simulink model "CM455A_Tauj0CfgAndUse"  (R2013b)
settings: Solver=FixedStepDiscrete  SolverMode=SingleTasking  StartTime=0.0  StopTime=1  FixedStep=0.0005  RelTol=1e-3
values from neighbouring files (symbols this model uses):
  PHAONTIMEASDMAX_NANOSEC_U32 = DataDict.Constant    [CM455A_Tauj0CfgAndUse_DataDict.m]
  TAUJ0TIPERCNT_NANOSECPERCNT_U15P1 = DataDict.Constant    [CM455A_Tauj0CfgAndUse_DataDict.m]
undefined symbols (not defined in the file or in its folder): sigbuilder_block
libraries: simulink x3, NxtrLim x3
settings Model: ModifiedHistory=Rev 008: Updated model to Matlab 2013B, added comments to show requirement linkage  Creator=nz3zln  LastModifiedBy=FZG88Y
settings SolverCC: AutoInsertRateTranBlk=on  InsertRTBMode=Always
settings DataIOCC: LimitDataPoints=off  SaveFormat=Structure  ReturnWorkspaceOutputs=on
settings OptimizationCC: BlockReduction=off  InlineParams=on  ZeroExternalMemoryAtStartup=off  ZeroInternalMemoryAtStartup=off  OptimizeModelRefInitCode=on  LifeSpan=1
settings DebuggingCC: SignalInfNanChecking=error  SignalRangeChecking=warning  UnderspecifiedInitializationDetection=Simplified  SolverPrmCheckMsg=error  InheritedTsInSrcMsg=error  DiscreteInheritContinuousMsg=error  SingleTaskRateTransMsg=error  TasksWithSamePriorityMsg=error  SigSpecEnsureSampleTimeMsg=error  CheckMatrixSingularityMsg=error  ParameterUnderflowMsg=error  ParameterPrecisionLossMsg=error  ParameterTunabilityLossMsg=error  FixptConstUnderflowMsg=warning  FixptConstOverflowMsg=warning  VectorMatrixConversionMsg=error  SignalLabelMismatchMsg=error  UnconnectedInputMsg=error  UnconnectedOutputMsg=error  UnconnectedLineMsg=error  SFcnCompatibilityMsg=error  UniqueDataStoreMsg=warning  BusObjectLabelMismatch=error  RootOutportRequireBusObject=error  AssertControl=DisableAll  ModelReferenceIOMsg=error  ModelReferenceVersionMismatchMessage=warning  ModelReferenceIOMismatchMessage=error  ModelReferenceCSMismatchMessage=warning  ModelReferenceDataLoggingMessage=error  StateNameClashWarn=warning  StrictBusMsg=ErrorOnBusTreatedAsVector  NonBusSignalsTreatedAsBus=error  SFUnexpectedBacktrackingDiag=error  SFInvalidInputDataAccessInChartInitDiag=error  SFNoUnconditionalDefaultTransitionDiag=error  SFTransitionOutsideNaturalParentDiag=error  SFUnconditionalTransitionShadowingDiag=error  SFUndirectedBroadcastEventsDiag=error
settings ModelReferenceCC: ModelReferenceNumInstancesAllowed=Single
settings RTWCC: SystemTargetFile=autosar.tlc  GenCodeOnly=on  TemplateMakefile=ert_default_tmf  Description=AUTOSAR  GenerateReport=on  ProcessScript=autosar_make_rtw_hook  LaunchReport=on
settings CodeAppCC: GenerateComments=off  IgnoreCustomStorageClasses=off  CustomSymbolStrType=$N$R$M  CustomSymbolStrBlkIO=$N$M  SimulinkBlockComments=off
settings STFCustomTargetCC: ParMdlRefBuildCompliant=on  CompOptLevelCompliant=on  IncludeMdlTerminateFcn=off  CombineOutputUpdateFcns=on  SuppressErrorStatus=on  ERTFirstTimeCompliant=on  ERTCustomFileBanners=on  SupportNonFinite=off  SupportComplex=off  SupportContinuousTime=off  SupportNonInlinedSFcns=off  MATLABClassNameForMDSCustomization=Simulink.SoftwareTarget.ERTCustomization  AutosarCompliant=on  GRTInterface=off  SystemTargetFile=autosar.tlc
settings ERTTargetCC: CodeReplacementLibrary=ANSI_C  ConcurrentExecutionCompliant=off  IncludeMdlTerminateFcn=off  SuppressErrorStatus=on  SupportNonFinite=off  SupportComplex=off  ModelStepFunctionPrototypeControlCompliant=off  CPPClassGenCompliant=off  AutosarCompliant=on  InlinedParameterPlacement=NonHierarchical  ERTCustomFileTemplate=example_file_process.tlc  EnableUserReplacementTypes=on

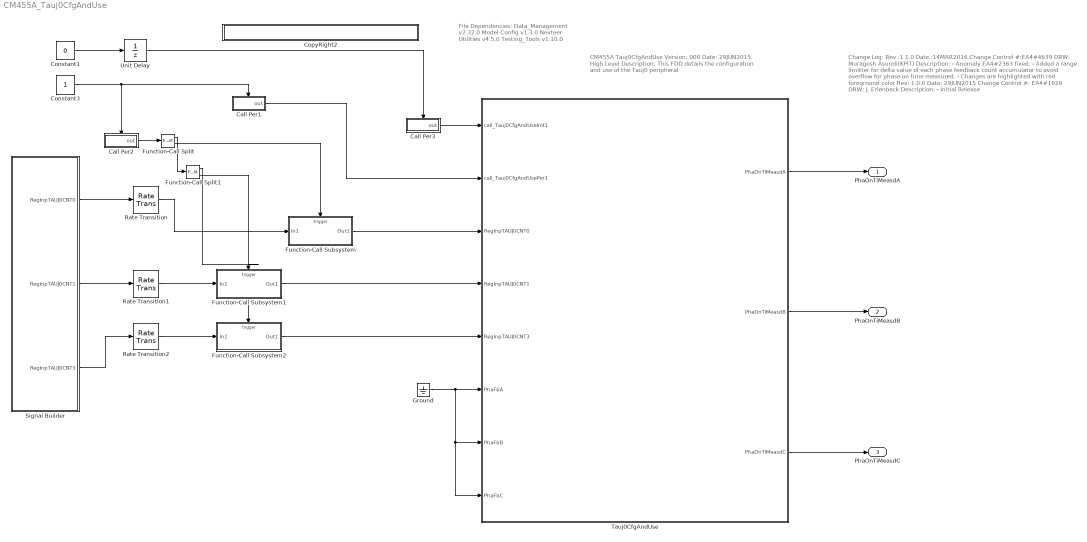
== system CM455A_Tauj0CfgAndUse ==
  note: CM455A Tauj0CfgAndUse
      |
      | Version: 000
      | Date: 29JUN2015
      |
      | High Level Description:
      | This FDD details the configuration and use of the Tauj0
      | peripheral
  note: Change Log:
      | Rev :1.1.0
      | Date :14MAR2016
      | Change Control #:EA4#4639
      | DRW: Muragesh Asundi(KPIT)
      | Description:
      | - Anomaly EA4#2363 fixed.
      | - Added a range limitter for delta value of each phase
      |  feedback count accumulator to avoid overflow for phase on time measured.
      | - Changes are highlighted with red foreground color
      |
      | Rev: 1.0.0
      | Date: 29JUN2015
      | Change Control #: EA4#1928
      | DRW: J. Erlenbeck
      | Description:
      | - Initial Release
  note: File Dependencies:
      | Data_Management v2.32.0
      | Model Config v1.3.0
      | Nexteer Utilities v4.5.0
      | Testing_Tools v1.10.0
  Call Per1 : Subsystem  TreatAsAtomicUnit=on
  Call Per2 : Subsystem  TreatAsAtomicUnit=on
  Call Per3 : Subsystem  TreatAsAtomicUnit=on
  Constant1 : Constant  Value=0  OutDataTypeStr=int8
  Constant3 : Constant  OutDataTypeStr=int8
  CopyRight2 : Subsystem  Description=|  mask(Copyright Information){none=on}
      | Copyright info block.                                               
      |                                                                     
      | Place copyright information at the top of every subsystem in design.
      mask prompts: none "No parameters"
      mask help: Place copyright information at the top of every subsystem in design.
      mask Display:
      | NxtrConf = 'Nexteer Confidential';
      | 
      | sys = bdroot; %handle for the current model ("system")
      | first = get_param(sys,'Created');
      | first = first(end-3:end);  %year is last four digits
      | 
      | last = get_param(sys,'LastModifiedDate');
      | if isempty(last)
      |     last = datestr(now,'yyyy');
      | else
      |     last = last(end-3:end);
      | end
      | 
      | if strcmp(first,last)
      |     fprintf('%s -- Copyright %s Nexteer',NxtrConf,first)
      | else
      |     fprintf('%s -- %s%s- %s Nexteer',NxtrConf,char(169),first,last)
      | end
  Function-Call Split : FunctionCallSplit
  Function-Call Split1 : FunctionCallSplit
  Function-Call Subsystem : Subsystem  TreatAsAtomicUnit=on
  Function-Call Subsystem1 : Subsystem  TreatAsAtomicUnit=on
  Function-Call Subsystem2 : Subsystem  TreatAsAtomicUnit=on
  Ground : Ground
  Rate Transition : RateTransition
  Rate Transition1 : RateTransition
  Rate Transition2 : RateTransition
  Signal Builder : Subsystem  Tag=STV Subsys  LoadFcn=sigbuilder_block('load');  StartFcn=sigbuilder_block('start');  StopFcn=sigbuilder_block('stop');  ClipboardFcn=sigbuilder_block('clipboard');  mask(Sigbuilder block){}
      mask help: Simulink:masks:SigbuilderBlock_MD
      mask init:
      | if ~strcmp(get_param(bdroot(gcbh),'SimulationStatus'),'stopped') tuvar = sigbuilder_block('maskInit'); end
      settings: CopyFcn=sigbuilder_block('copy');  DeleteFcn=sigbuilder_block('delete');  ModelCloseFcn=sigbuilder_block('modelClose');  PreSaveFcn=sigbuilder_block('preSave');  PauseFcn=sigbuilder_block('pause');  ContinueFcn=sigbuilder_block('continue');  NameChangeFcn=sigbuilder_block('namechange');  OpenFcn=sigbuilder_block('open',[0 124.5 635.25 388.5 ]);  CloseFcn=sigbuilder_block('close');
      mask Display: plot(0, 0, 100, 100,[2, 2, 32, 32, 2], [68, 8, 8, 68, 68],[32, 2], [38, 38], [32, 19, 2],[53, 60, 44], [32, 17, 17, 2],[16, 16, 31, 31]);txt = getActiveGroup(gcbh);text(2, 100, txt,'verticalAlignment', 'top');
  Tauj0CfgAndUse : Subsystem
  Unit Delay : UnitDelay  InitialCondition=1  SampleTime=-1
  PhaOnTiMeasdA : Outport
  PhaOnTiMeasdB : Outport  Port=2
  PhaOnTiMeasdC : Outport  Port=3
  wires:
  Constant3/1 -> Call Per2/Enable, Call Per1/Enable
  Signal Builder/1(RegInpTAUJ0CNT0) -> Rate Transition/1
  Call Per1/1(out) -> Tauj0CfgAndUse/2(call_Tauj0CfgAndUsePer1)
  Function-Call Subsystem/1(Out1) -> Tauj0CfgAndUse/3(RegInpTAUJ0CNT0)
  Rate Transition/1 -> Function-Call Subsystem/1(In1)
  Signal Builder/2(RegInpTAUJ0CNT1) -> Rate Transition1/1
  Signal Builder/3(RegInpTAUJ0CNT3) -> Rate Transition2/1
  Rate Transition1/1 -> Function-Call Subsystem1/1(In1)
  Rate Transition2/1 -> Function-Call Subsystem2/1(In1)
  Call Per2/1(out) -> Function-Call Split/1
  Function-Call Split/2 -> Function-Call Subsystem/Trigger
  Function-Call Split/1 -> Function-Call Split1/1
  Function-Call Split1/2 -> Function-Call Subsystem1/Trigger
  Function-Call Split1/1 -> Function-Call Subsystem2/Trigger
  Function-Call Subsystem1/1(Out1) -> Tauj0CfgAndUse/4(RegInpTAUJ0CNT1)
  Function-Call Subsystem2/1(Out1) -> Tauj0CfgAndUse/5(RegInpTAUJ0CNT3)
  Constant1/1 -> Unit Delay/1
  Unit Delay/1 -> Call Per3/Enable
  Call Per3/1(out) -> Tauj0CfgAndUse/1(call_Tauj0CfgAndUseInit1)
  Ground/1 -> Tauj0CfgAndUse/8(PhaFbC), Tauj0CfgAndUse/7(PhaFbB), Tauj0CfgAndUse/6(PhaFbA)
  Tauj0CfgAndUse/1(PhaOnTiMeasdA) -> PhaOnTiMeasdA/1
  Tauj0CfgAndUse/2(PhaOnTiMeasdB) -> PhaOnTiMeasdB/1
  Tauj0CfgAndUse/3(PhaOnTiMeasdC) -> PhaOnTiMeasdC/1

== system CM455A_Tauj0CfgAndUse/Call Per1 ==
  Enable : EnablePort
  Function Call Trigger : simulink/Ports & Subsystems/Function-Call Generator  RequirementInfo={} %GIDa_6dd05ab1_f91b_4d7a_a0ec_1170d213fa7b  sample_time=0.002  numberOfIterations=1
  out : Outport
  wires:
  Function Call Trigger/1 -> out/1

== system CM455A_Tauj0CfgAndUse/Call Per2 ==
  Enable : EnablePort
  Function Call Trigger : simulink/Ports & Subsystems/Function-Call Generator  RequirementInfo={} %GIDa_ae766dae_e1c3_424a_a7dd_99da62b4e21f  sample_time=0.0005  numberOfIterations=1
  out : Outport
  wires:
  Function Call Trigger/1 -> out/1

== system CM455A_Tauj0CfgAndUse/Call Per3 ==
  Enable : EnablePort
  Function Call Trigger : simulink/Ports & Subsystems/Function-Call Generator  RequirementInfo={} %GIDa_4dbf052b_4973_407d_b675_b3a9817a3516  sample_time=0.002  numberOfIterations=1
  out : Outport
  wires:
  Function Call Trigger/1 -> out/1

== system CM455A_Tauj0CfgAndUse/CopyRight2 ==

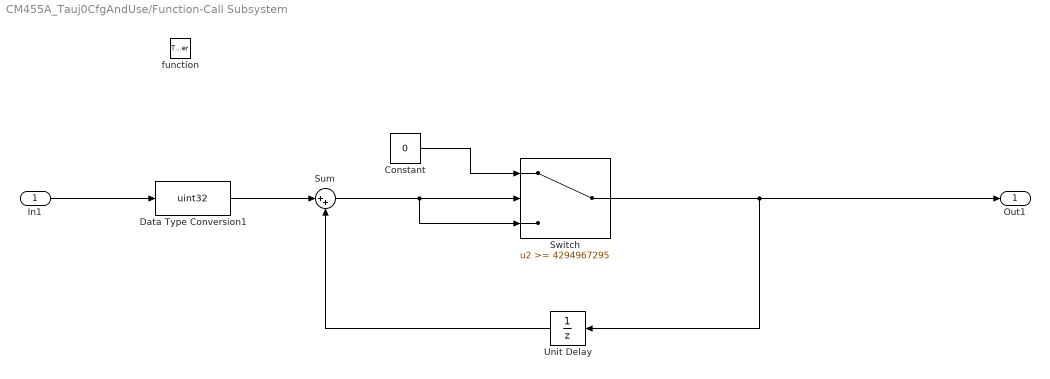
== system CM455A_Tauj0CfgAndUse/Function-Call Subsystem ==
  In1 : Inport
  function : TriggerPort  TriggerType=function-call
  Constant : Constant  Value=0  OutDataTypeStr=uint16
  Data Type Conversion1 : DataTypeConversion  OutDataTypeStr=uint32  RndMeth=Nearest
  Sum : Sum  Inputs=|++
  Switch : Switch  Threshold=4294967295
  Unit Delay : UnitDelay  SampleTime=-1
  Out1 : Outport
  wires:
  Constant/1 -> Switch/1
  Sum/1 -> Switch/3, Switch/2
  Data Type Conversion1/1 -> Sum/1
  Switch/1 -> Out1/1, Unit Delay/1
  Unit Delay/1 -> Sum/2
  In1/1 -> Data Type Conversion1/1

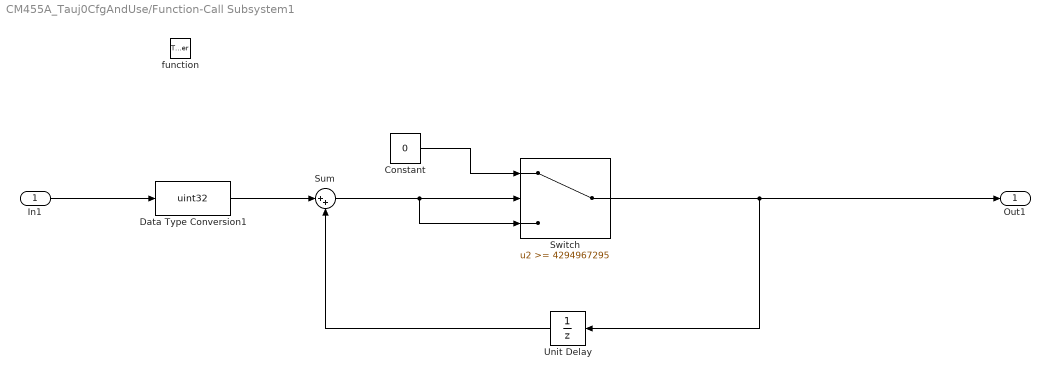
== system CM455A_Tauj0CfgAndUse/Function-Call Subsystem1 ==
  In1 : Inport
  function : TriggerPort  TriggerType=function-call
  Constant : Constant  Value=0  OutDataTypeStr=uint16
  Data Type Conversion1 : DataTypeConversion  OutDataTypeStr=uint32  RndMeth=Nearest
  Sum : Sum  Inputs=|++
  Switch : Switch  Threshold=4294967295
  Unit Delay : UnitDelay  SampleTime=-1
  Out1 : Outport
  wires:
  In1/1 -> Data Type Conversion1/1
  Unit Delay/1 -> Sum/2
  Switch/1 -> Unit Delay/1, Out1/1
  Data Type Conversion1/1 -> Sum/1
  Sum/1 -> Switch/2, Switch/3
  Constant/1 -> Switch/1

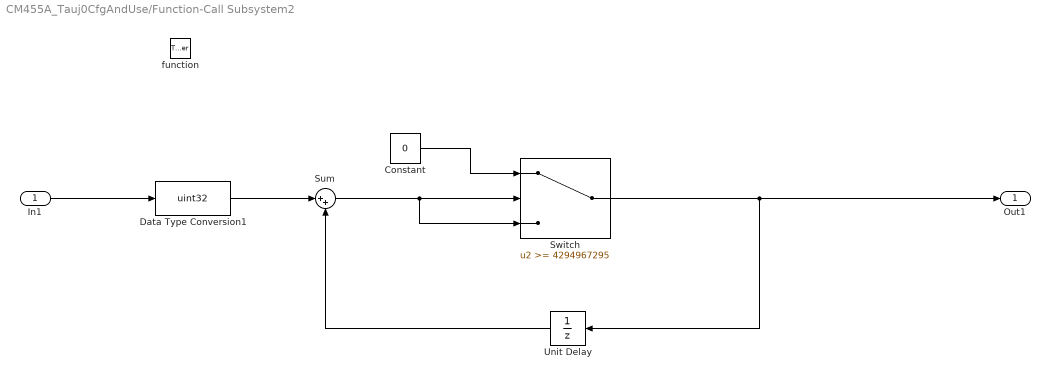
== system CM455A_Tauj0CfgAndUse/Function-Call Subsystem2 ==
  In1 : Inport
  function : TriggerPort  TriggerType=function-call
  Constant : Constant  Value=0  OutDataTypeStr=uint16
  Data Type Conversion1 : DataTypeConversion  OutDataTypeStr=uint32  RndMeth=Nearest
  Sum : Sum  Inputs=|++
  Switch : Switch  Threshold=4294967295
  Unit Delay : UnitDelay  SampleTime=-1
  Out1 : Outport
  wires:
  Constant/1 -> Switch/1
  Sum/1 -> Switch/3, Switch/2
  Data Type Conversion1/1 -> Sum/1
  Switch/1 -> Out1/1, Unit Delay/1
  Unit Delay/1 -> Sum/2
  In1/1 -> Data Type Conversion1/1

== system CM455A_Tauj0CfgAndUse/Signal Builder ==
  Demux : Demux  Tag=STV Demux  Outputs=3
  FromWs : FromWorkspace  Tag=STV FromWs  VariableName=tuvar  SampleTime=0
      SigBuilderData=|
      | common.afterFinalStr = 'Extrapolate'
      | common.sampleTime = 0
      | dataSet.timeRange = [0 2]
      | dataSet.name = 'Group 1'
      | sbobj.Groups.Name = 'Group 1'
      | sbobj.Groups.Signals(1).Name = 'RegInpTAUJ0CNT0'
      | sbobj.Groups.Signals(1).XData = [0 0.00125628140704 0.00251256281407 0.00376884422111 0.00502512562814 0.00628140703518 0.00753768844221 0.00879396984925 0.0100502512563 0.0113065326633 0.0125628140704 0.0138190954774 ... (1593 elements, 1x1593)]
      | sbobj.Groups.Signals(1).YData = [5000000 5157842.74882 5315528.15656 5472899.03897 5629798.52534 5786070.21484 5941558.33245 6096107.88424 6249564.81185 6401776.14609 6552590.15937 6701856.51702 ... (1593 elements, 1x1593)]
      | sbobj.Groups.Signals(2).Name = 'RegInpTAUJ0CNT1'
      | sbobj.Groups.Signals(2).XData = [0 0.5 0.5 1 1 1.5 1.5 2]
      | sbobj.Groups.Signals(2).YData = [0 4000000 0 4000000 0 4000000 0 4000000]
      | sbobj.Groups.Signals(3).Name = 'RegInpTAUJ0CNT3'
      | sbobj.Groups.Signals(3).XData = [0 0.0833333333333 0.0833333333333 0.2 0.2 0.416666666667 0.416666666667 0.514 0.514 0.966 0.966 1 1 1.298 1.298 1.33333333333 1.33333333333 1.598 1.598 1.66666666667 1.66666666667 1.946 1.946 2]
      | sbobj.Groups.Signals(3).YData = [10000000 10000000 0 0 10000000 10000000 0 0 10000000 10000000 0 0 10000000 10000000 0 0 10000000 10000000 0 0 10000000 10000000 0 0]
      | sbobj.Groups.TimeRange = [0 2]
  RegInpTAUJ0CNT0 : Outport  Tag=STV Outport
  RegInpTAUJ0CNT1 : Outport  Tag=STV Outport  Port=2
  RegInpTAUJ0CNT3 : Outport  Tag=STV Outport  Port=3
  wires:
  FromWs/1 -> Demux/1
  Demux/1 -> RegInpTAUJ0CNT0/1
  Demux/2 -> RegInpTAUJ0CNT1/1
  Demux/3 -> RegInpTAUJ0CNT3/1

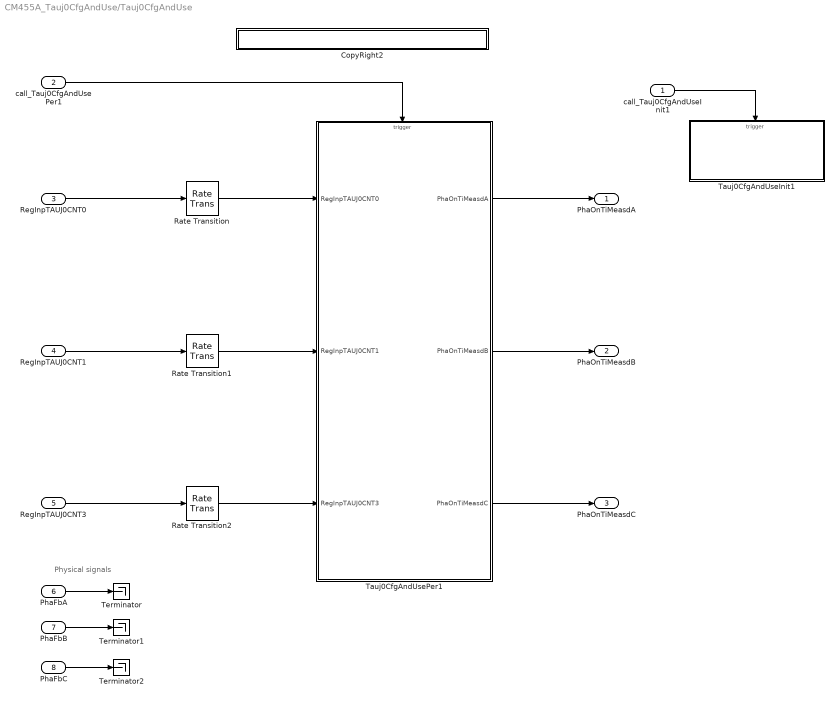
== system CM455A_Tauj0CfgAndUse/Tauj0CfgAndUse ==
  note: Physical signals
  call_Tauj0CfgAndUseInit1 : Inport  RequirementInfo={} %GIDa_c75e8815_b602_4250_97f2_eeb5dd1c39d1
  call_Tauj0CfgAndUsePer1 : Inport  RequirementInfo={} %GIDa_468d2479_6710_42ce_bd19_b69834ab6306  Port=2
  RegInpTAUJ0CNT0 : Inport  Port=3
  RegInpTAUJ0CNT1 : Inport  Port=4
  RegInpTAUJ0CNT3 : Inport  RequirementInfo={} %GIDa_84fb02b3_72b4_4e28_a17f_e99f7297de00  Port=5
  PhaFbA : Inport  Port=6
  PhaFbB : Inport  Port=7
  PhaFbC : Inport  Port=8
  CopyRight2 : Subsystem  Description=|  mask(Copyright Information){none=on}
      | Copyright info block.                                               
      |                                                                     
      | Place copyright information at the top of every subsystem in design.
      mask prompts: none "No parameters"
      mask help: Place copyright information at the top of every subsystem in design.
      mask Display:
      | NxtrConf = 'Nexteer Confidential';
      | 
      | sys = bdroot; %handle for the current model ("system")
      | first = get_param(sys,'Created');
      | first = first(end-3:end);  %year is last four digits
      | 
      | last = get_param(sys,'LastModifiedDate');
      | if isempty(last)
      |     last = datestr(now,'yyyy');
      | else
      |     last = last(end-3:end);
      | end
      | 
      | if strcmp(first,last)
      |     fprintf('%s -- Copyright %s Nexteer',NxtrConf,first)
      | else
      |     fprintf('%s -- %s%s- %s Nexteer',NxtrConf,char(169),first,last)
      | end
  Rate Transition : RateTransition
  Rate Transition1 : RateTransition
  Rate Transition2 : RateTransition
  Tauj0CfgAndUseInit1 : Subsystem  TreatAsAtomicUnit=on
  Tauj0CfgAndUsePer1 : Subsystem  TreatAsAtomicUnit=on
  Terminator : Terminator
  Terminator1 : Terminator
  Terminator2 : Terminator
  PhaOnTiMeasdA : Outport
  PhaOnTiMeasdB : Outport  Port=2
  PhaOnTiMeasdC : Outport  Port=3
  wires:
  call_Tauj0CfgAndUsePer1/1 -> Tauj0CfgAndUsePer1/Trigger
  RegInpTAUJ0CNT0/1 -> Rate Transition/1
  RegInpTAUJ0CNT1/1 -> Rate Transition1/1
  RegInpTAUJ0CNT3/1 -> Rate Transition2/1
  Rate Transition/1 -> Tauj0CfgAndUsePer1/1(RegInpTAUJ0CNT0)
  Rate Transition1/1 -> Tauj0CfgAndUsePer1/2(RegInpTAUJ0CNT1)
  Rate Transition2/1 -> Tauj0CfgAndUsePer1/3(RegInpTAUJ0CNT3)
  Tauj0CfgAndUsePer1/1(PhaOnTiMeasdA) -> PhaOnTiMeasdA/1
  Tauj0CfgAndUsePer1/2(PhaOnTiMeasdB) -> PhaOnTiMeasdB/1
  Tauj0CfgAndUsePer1/3(PhaOnTiMeasdC) -> PhaOnTiMeasdC/1
  call_Tauj0CfgAndUseInit1/1 -> Tauj0CfgAndUseInit1/Trigger
  PhaFbA/1 -> Terminator/1
  PhaFbB/1 -> Terminator1/1
  PhaFbC/1 -> Terminator2/1

== system CM455A_Tauj0CfgAndUse/Tauj0CfgAndUse/CopyRight2 ==

== system CM455A_Tauj0CfgAndUse/Tauj0CfgAndUse/Tauj0CfgAndUseInit1 ==
  note: Initialize the Tauj0 registers per
      | CM455A_Tauj0CfgAndUse_RegisterConfiguration.xlsm.  Initialize in order by row, top to bottom.
  function : TriggerPort  TriggerType=function-call
  CopyRight2 : Subsystem  Description=|  mask(Copyright Information){none=on}
      | Copyright info block.                                               
      |                                                                     
      | Place copyright information at the top of every subsystem in design.
      mask prompts: none "No parameters"
      mask help: Place copyright information at the top of every subsystem in design.
      mask Display:
      | NxtrConf = 'Nexteer Confidential';
      | 
      | sys = bdroot; %handle for the current model ("system")
      | first = get_param(sys,'Created');
      | first = first(end-3:end);  %year is last four digits
      | 
      | last = get_param(sys,'LastModifiedDate');
      | if isempty(last)
      |     last = datestr(now,'yyyy');
      | else
      |     last = last(end-3:end);
      | end
      | 
      | if strcmp(first,last)
      |     fprintf('%s -- Copyright %s Nexteer',NxtrConf,first)
      | else
      |     fprintf('%s -- %s%s- %s Nexteer',NxtrConf,char(169),first,last)
      | end

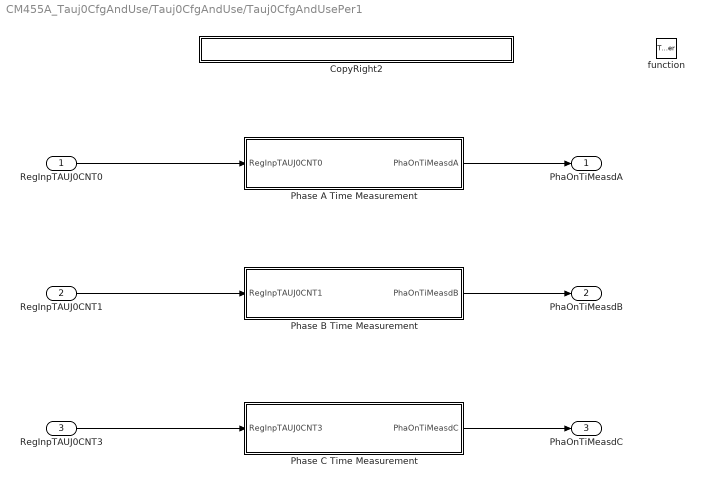
== system CM455A_Tauj0CfgAndUse/Tauj0CfgAndUse/Tauj0CfgAndUsePer1 ==
  RegInpTAUJ0CNT0 : Inport
  RegInpTAUJ0CNT1 : Inport  Port=2
  RegInpTAUJ0CNT3 : Inport  RequirementInfo={} %GIDa_d2e38bc4_d7b3_4726_bec9_8ac60b17d0ae  Port=3
  function : TriggerPort  TriggerType=function-call
  CopyRight2 : Subsystem  Description=|  mask(Copyright Information){none=on}
      | Copyright info block.                                               
      |                                                                     
      | Place copyright information at the top of every subsystem in design.
      mask prompts: none "No parameters"
      mask help: Place copyright information at the top of every subsystem in design.
      mask Display:
      | NxtrConf = 'Nexteer Confidential';
      | 
      | sys = bdroot; %handle for the current model ("system")
      | first = get_param(sys,'Created');
      | first = first(end-3:end);  %year is last four digits
      | 
      | last = get_param(sys,'LastModifiedDate');
      | if isempty(last)
      |     last = datestr(now,'yyyy');
      | else
      |     last = last(end-3:end);
      | end
      | 
      | if strcmp(first,last)
      |     fprintf('%s -- Copyright %s Nexteer',NxtrConf,first)
      | else
      |     fprintf('%s -- %s%s- %s Nexteer',NxtrConf,char(169),first,last)
      | end
  Phase A Time Measurement : Subsystem  RequirementInfo="{'linktype_rmi_doors' '0000cf4a (/ESG Group/FDD Module Requirements/EA4 Specific/CM455A_Tauj0CfgAndMeas)' '#CM455A_87' 'true' 'REQ:  CM455A_87' '' } %GIDa_7041a376_39d9_4031_9ce0_54f885feabcb"  TreatAsAtomicUnit=on
  Phase B Time Measurement : Subsystem  RequirementInfo="{'linktype_rmi_doors' '0000cf4a (/ESG Group/FDD Module Requirements/EA4 Specific/CM455A_Tauj0CfgAndMeas)' '#CM455A_95' 'true' 'REQ:  CM455A_95' '' } %GIDa_2958352a_abfa_49fb_ac22_38a600953ff5"  TreatAsAtomicUnit=on
  Phase C Time Measurement : Subsystem  RequirementInfo="{'linktype_rmi_doors' '0000cf4a (/ESG Group/FDD Module Requirements/EA4 Specific/CM455A_Tauj0CfgAndMeas)' '#CM455A_96' 'true' 'REQ:  CM455A_96' '' } %GIDa_b9e937c9_f0a4_435c_8980_887e05030cab"  TreatAsAtomicUnit=on
  PhaOnTiMeasdA : Outport
  PhaOnTiMeasdB : Outport  Port=2
  PhaOnTiMeasdC : Outport  Port=3
  wires:
  Phase A Time Measurement/1(PhaOnTiMeasdA) -> PhaOnTiMeasdA/1
  RegInpTAUJ0CNT0/1 -> Phase A Time Measurement/1(RegInpTAUJ0CNT0)
  Phase B Time Measurement/1(PhaOnTiMeasdB) -> PhaOnTiMeasdB/1
  RegInpTAUJ0CNT1/1 -> Phase B Time Measurement/1(RegInpTAUJ0CNT1)
  RegInpTAUJ0CNT3/1 -> Phase C Time Measurement/1(RegInpTAUJ0CNT3)
  Phase C Time Measurement/1(PhaOnTiMeasdC) -> PhaOnTiMeasdC/1

== system CM455A_Tauj0CfgAndUse/Tauj0CfgAndUse/Tauj0CfgAndUseInit1/CopyRight2 ==

== system CM455A_Tauj0CfgAndUse/Tauj0CfgAndUse/Tauj0CfgAndUsePer1/CopyRight2 ==

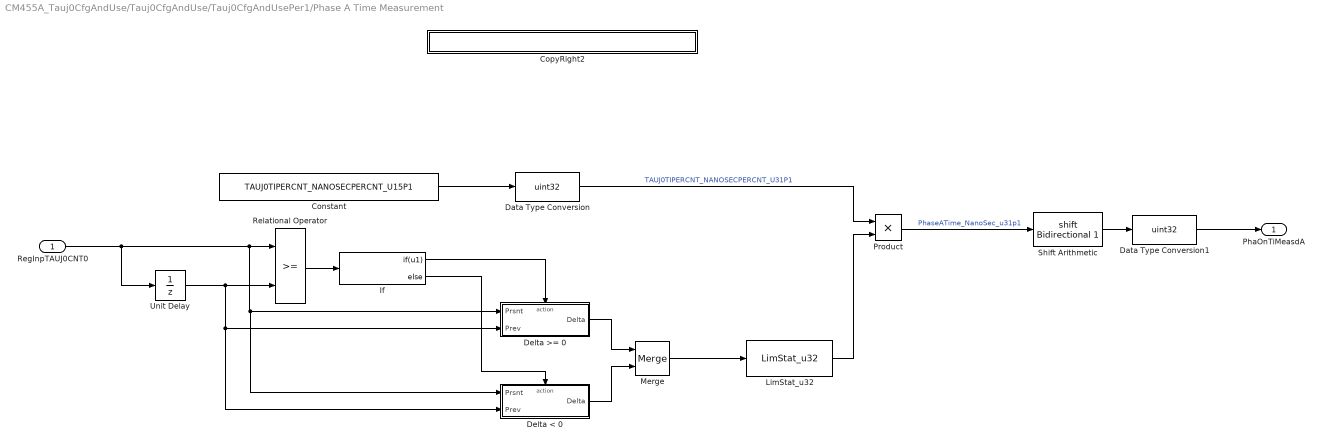
== system CM455A_Tauj0CfgAndUse/Tauj0CfgAndUse/Tauj0CfgAndUsePer1/Phase A Time Measurement ==
  RegInpTAUJ0CNT0 : Inport
  Constant : Constant  Value=TAUJ0TIPERCNT_NANOSECPERCNT_U15P1
  CopyRight2 : Subsystem  Description=|  mask(Copyright Information){none=on}
      | Copyright info block.                                               
      |                                                                     
      | Place copyright information at the top of every subsystem in design.
      mask prompts: none "No parameters"
      mask help: Place copyright information at the top of every subsystem in design.
      mask Display:
      | NxtrConf = 'Nexteer Confidential';
      | 
      | sys = bdroot; %handle for the current model ("system")
      | first = get_param(sys,'Created');
      | first = first(end-3:end);  %year is last four digits
      | 
      | last = get_param(sys,'LastModifiedDate');
      | if isempty(last)
      |     last = datestr(now,'yyyy');
      | else
      |     last = last(end-3:end);
      | end
      | 
      | if strcmp(first,last)
      |     fprintf('%s -- Copyright %s Nexteer',NxtrConf,first)
      | else
      |     fprintf('%s -- %s%s- %s Nexteer',NxtrConf,char(169),first,last)
      | end
  Data Type Conversion : DataTypeConversion  OutDataTypeStr=uint32
  Data Type Conversion1 : DataTypeConversion  OutDataTypeStr=uint32
  Delta < 0 : Subsystem  TreatAsAtomicUnit=on
  Delta >= 0 : Subsystem  TreatAsAtomicUnit=on
  If : If  IfExpression=u1
  LimStat_u32 : NxtrLim/LimStat_u32  LoLim=PHAFBDELTACNTMIN_CNT_U32  HiLim=PHAFBDELTACNTMAX_CNT_U32
      settings: AttributesFormatString=|
      | Low Limit: %<LoLim>
      | High Limit:%<HiLim>
  Merge : Merge
  Product : Product
  Relational Operator : RelationalOperator  OutDataTypeStr=boolean
  Shift Arithmetic : ArithShift  BitShiftNumber=1
  Unit Delay : UnitDelay  SampleTime=-1  StateName=PhaOnTiCntrAPrev  StateMustResolveToSignalObject=on
      settings: AttributesFormatString=|
      | State Variable:
      | %<StateName>
  PhaOnTiMeasdA : Outport
  wires:
  Unit Delay/1 -> Delta < 0/2(Prev), Delta >= 0/2(Prev), Relational Operator/2
  Constant/1 -> Data Type Conversion/1
  Data Type Conversion/1 -> Product/1  "TAUJ0TIPERCNT_NANOSECPERCNT_U31P1"
  Shift Arithmetic/1 -> Data Type Conversion1/1
  Data Type Conversion1/1 -> PhaOnTiMeasdA/1
  RegInpTAUJ0CNT0/1 -> Delta < 0/1(Prsnt), Delta >= 0/1(Prsnt), Relational Operator/1, Unit Delay/1
  Product/1 -> Shift Arithmetic/1  "PhaseATime_NanoSec_u31p1"
  Relational Operator/1 -> If/1
  If/1 -> Delta >= 0/Action
  If/2 -> Delta < 0/Action
  LimStat_u32/1 -> Product/2
  Delta >= 0/1(Delta) -> Merge/1
  Delta < 0/1(Delta) -> Merge/2
  Merge/1 -> LimStat_u32/1

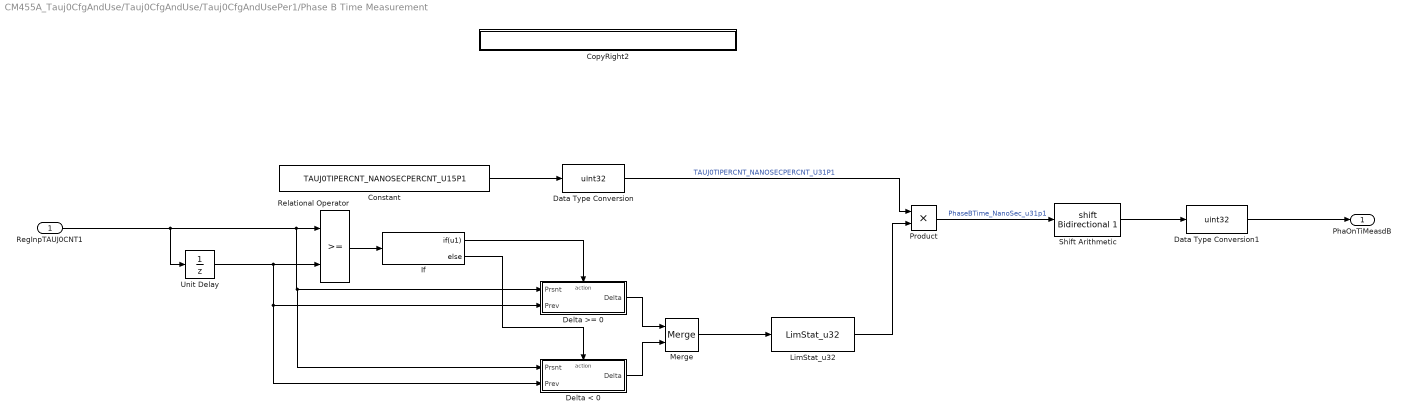
== system CM455A_Tauj0CfgAndUse/Tauj0CfgAndUse/Tauj0CfgAndUsePer1/Phase B Time Measurement ==
  RegInpTAUJ0CNT1 : Inport
  Constant : Constant  Value=TAUJ0TIPERCNT_NANOSECPERCNT_U15P1
  CopyRight2 : Subsystem  Description=|  mask(Copyright Information){none=on}
      | Copyright info block.                                               
      |                                                                     
      | Place copyright information at the top of every subsystem in design.
      mask prompts: none "No parameters"
      mask help: Place copyright information at the top of every subsystem in design.
      mask Display:
      | NxtrConf = 'Nexteer Confidential';
      | 
      | sys = bdroot; %handle for the current model ("system")
      | first = get_param(sys,'Created');
      | first = first(end-3:end);  %year is last four digits
      | 
      | last = get_param(sys,'LastModifiedDate');
      | if isempty(last)
      |     last = datestr(now,'yyyy');
      | else
      |     last = last(end-3:end);
      | end
      | 
      | if strcmp(first,last)
      |     fprintf('%s -- Copyright %s Nexteer',NxtrConf,first)
      | else
      |     fprintf('%s -- %s%s- %s Nexteer',NxtrConf,char(169),first,last)
      | end
  Data Type Conversion : DataTypeConversion  OutDataTypeStr=uint32
  Data Type Conversion1 : DataTypeConversion  OutDataTypeStr=uint32
  Delta < 0 : Subsystem  TreatAsAtomicUnit=on
  Delta >= 0 : Subsystem  TreatAsAtomicUnit=on
  If : If  IfExpression=u1
  LimStat_u32 : NxtrLim/LimStat_u32  LoLim=PHAFBDELTACNTMIN_CNT_U32  HiLim=PHAFBDELTACNTMAX_CNT_U32
      settings: AttributesFormatString=|
      | Low Limit: %<LoLim>
      | High Limit:%<HiLim>
  Merge : Merge
  Product : Product
  Relational Operator : RelationalOperator  OutDataTypeStr=boolean
  Shift Arithmetic : ArithShift  BitShiftNumber=1
  Unit Delay : UnitDelay  SampleTime=-1  StateName=PhaOnTiCntrBPrev  StateMustResolveToSignalObject=on
      settings: AttributesFormatString=|
      | State Variable:
      | %<StateName>
  PhaOnTiMeasdB : Outport
  wires:
  Shift Arithmetic/1 -> Data Type Conversion1/1
  Product/1 -> Shift Arithmetic/1  "PhaseBTime_NanoSec_u31p1"
  Data Type Conversion/1 -> Product/1  "TAUJ0TIPERCNT_NANOSECPERCNT_U31P1"
  Constant/1 -> Data Type Conversion/1
  Data Type Conversion1/1 -> PhaOnTiMeasdB/1
  Unit Delay/1 -> Delta < 0/2(Prev), Delta >= 0/2(Prev), Relational Operator/2
  RegInpTAUJ0CNT1/1 -> Delta < 0/1(Prsnt), Delta >= 0/1(Prsnt), Relational Operator/1, Unit Delay/1
  Relational Operator/1 -> If/1
  If/1 -> Delta >= 0/Action
  If/2 -> Delta < 0/Action
  LimStat_u32/1 -> Product/2
  Delta >= 0/1(Delta) -> Merge/1
  Delta < 0/1(Delta) -> Merge/2
  Merge/1 -> LimStat_u32/1

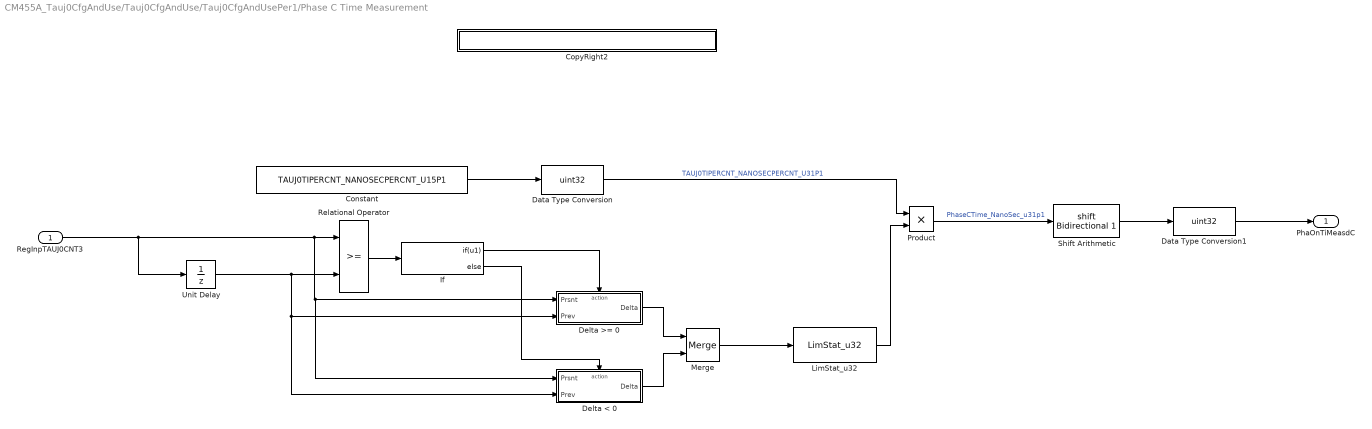
== system CM455A_Tauj0CfgAndUse/Tauj0CfgAndUse/Tauj0CfgAndUsePer1/Phase C Time Measurement ==
  RegInpTAUJ0CNT3 : Inport
  Constant : Constant  Value=TAUJ0TIPERCNT_NANOSECPERCNT_U15P1
  CopyRight2 : Subsystem  Description=|  mask(Copyright Information){none=on}
      | Copyright info block.                                               
      |                                                                     
      | Place copyright information at the top of every subsystem in design.
      mask prompts: none "No parameters"
      mask help: Place copyright information at the top of every subsystem in design.
      mask Display:
      | NxtrConf = 'Nexteer Confidential';
      | 
      | sys = bdroot; %handle for the current model ("system")
      | first = get_param(sys,'Created');
      | first = first(end-3:end);  %year is last four digits
      | 
      | last = get_param(sys,'LastModifiedDate');
      | if isempty(last)
      |     last = datestr(now,'yyyy');
      | else
      |     last = last(end-3:end);
      | end
      | 
      | if strcmp(first,last)
      |     fprintf('%s -- Copyright %s Nexteer',NxtrConf,first)
      | else
      |     fprintf('%s -- %s%s- %s Nexteer',NxtrConf,char(169),first,last)
      | end
  Data Type Conversion : DataTypeConversion  OutDataTypeStr=uint32
  Data Type Conversion1 : DataTypeConversion  OutDataTypeStr=uint32
  Delta < 0 : Subsystem  TreatAsAtomicUnit=on
  Delta >= 0 : Subsystem  TreatAsAtomicUnit=on
  If : If  IfExpression=u1
  LimStat_u32 : NxtrLim/LimStat_u32  LoLim=PHAFBDELTACNTMIN_CNT_U32  HiLim=PHAFBDELTACNTMAX_CNT_U32
      settings: AttributesFormatString=|
      | Low Limit: %<LoLim>
      | High Limit:%<HiLim>
  Merge : Merge
  Product : Product
  Relational Operator : RelationalOperator  OutDataTypeStr=boolean
  Shift Arithmetic : ArithShift  BitShiftNumber=1
  Unit Delay : UnitDelay  SampleTime=-1  StateName=PhaOnTiCntrCPrev  StateMustResolveToSignalObject=on
      settings: AttributesFormatString=|
      | State Variable:
      | %<StateName>
  PhaOnTiMeasdC : Outport
  wires:
  Constant/1 -> Data Type Conversion/1
  Data Type Conversion/1 -> Product/1  "TAUJ0TIPERCNT_NANOSECPERCNT_U31P1"
  Product/1 -> Shift Arithmetic/1  "PhaseCTime_NanoSec_u31p1"
  Shift Arithmetic/1 -> Data Type Conversion1/1
  Data Type Conversion1/1 -> PhaOnTiMeasdC/1
  Unit Delay/1 -> Delta >= 0/2(Prev), Delta < 0/2(Prev), Relational Operator/2
  RegInpTAUJ0CNT3/1 -> Delta < 0/1(Prsnt), Delta >= 0/1(Prsnt), Relational Operator/1, Unit Delay/1
  Relational Operator/1 -> If/1
  If/1 -> Delta >= 0/Action
  If/2 -> Delta < 0/Action
  LimStat_u32/1 -> Product/2
  Delta >= 0/1(Delta) -> Merge/1
  Delta < 0/1(Delta) -> Merge/2
  Merge/1 -> LimStat_u32/1

== system CM455A_Tauj0CfgAndUse/Tauj0CfgAndUse/Tauj0CfgAndUsePer1/Phase A Time Measurement/CopyRight2 ==

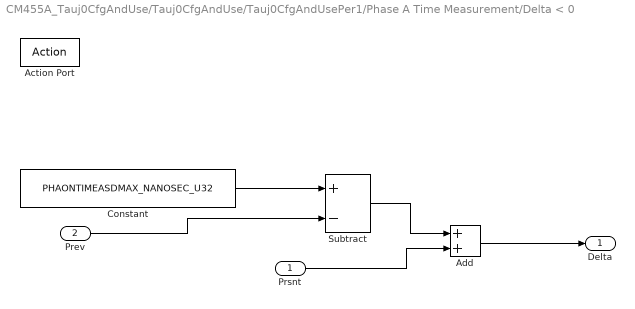
== system CM455A_Tauj0CfgAndUse/Tauj0CfgAndUse/Tauj0CfgAndUsePer1/Phase A Time Measurement/Delta < 0 ==
  Prsnt : Inport
  Prev : Inport  Port=2
  Action Port : ActionPort  ActionType=else
  Add : Sum
  Constant : Constant  Value=PHAONTIMEASDMAX_NANOSEC_U32
  Subtract : Sum  Inputs=+-
  Delta : Outport
  wires:
  Constant/1 -> Subtract/1
  Prev/1 -> Subtract/2
  Add/1 -> Delta/1
  Subtract/1 -> Add/1
  Prsnt/1 -> Add/2

== system CM455A_Tauj0CfgAndUse/Tauj0CfgAndUse/Tauj0CfgAndUsePer1/Phase A Time Measurement/Delta >= 0 ==
  Prsnt : Inport
  Prev : Inport  Port=2
  Action Port : ActionPort  ActionType=then
  Subtract : Sum  Inputs=+-
  Delta : Outport
  wires:
  Subtract/1 -> Delta/1
  Prsnt/1 -> Subtract/1
  Prev/1 -> Subtract/2

== system CM455A_Tauj0CfgAndUse/Tauj0CfgAndUse/Tauj0CfgAndUsePer1/Phase B Time Measurement/CopyRight2 ==

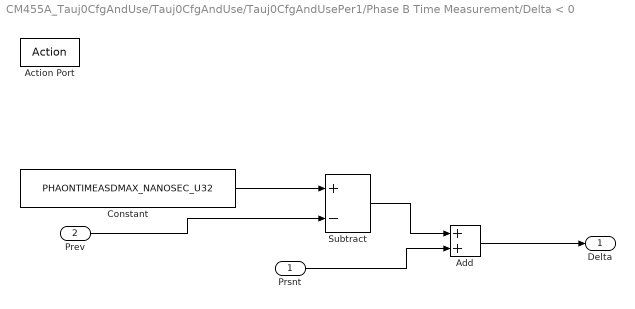
== system CM455A_Tauj0CfgAndUse/Tauj0CfgAndUse/Tauj0CfgAndUsePer1/Phase B Time Measurement/Delta < 0 ==
  Prsnt : Inport
  Prev : Inport  Port=2
  Action Port : ActionPort  ActionType=else
  Add : Sum
  Constant : Constant  Value=PHAONTIMEASDMAX_NANOSEC_U32
  Subtract : Sum  Inputs=+-
  Delta : Outport
  wires:
  Constant/1 -> Subtract/1
  Prev/1 -> Subtract/2
  Add/1 -> Delta/1
  Subtract/1 -> Add/1
  Prsnt/1 -> Add/2

== system CM455A_Tauj0CfgAndUse/Tauj0CfgAndUse/Tauj0CfgAndUsePer1/Phase B Time Measurement/Delta >= 0 ==
  Prsnt : Inport
  Prev : Inport  Port=2
  Action Port : ActionPort  ActionType=then
  Subtract : Sum  Inputs=+-
  Delta : Outport
  wires:
  Subtract/1 -> Delta/1
  Prsnt/1 -> Subtract/1
  Prev/1 -> Subtract/2

== system CM455A_Tauj0CfgAndUse/Tauj0CfgAndUse/Tauj0CfgAndUsePer1/Phase C Time Measurement/CopyRight2 ==

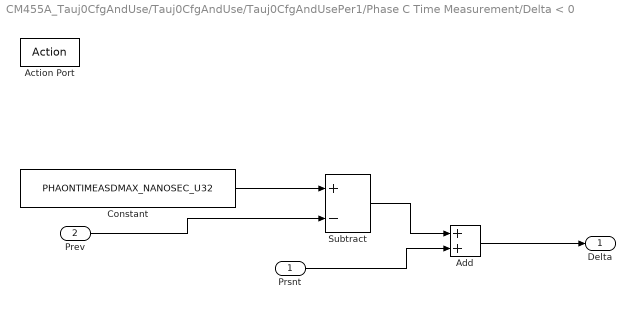
== system CM455A_Tauj0CfgAndUse/Tauj0CfgAndUse/Tauj0CfgAndUsePer1/Phase C Time Measurement/Delta < 0 ==
  Prsnt : Inport
  Prev : Inport  Port=2
  Action Port : ActionPort  ActionType=else
  Add : Sum
  Constant : Constant  Value=PHAONTIMEASDMAX_NANOSEC_U32
  Subtract : Sum  Inputs=+-
  Delta : Outport
  wires:
  Constant/1 -> Subtract/1
  Prev/1 -> Subtract/2
  Add/1 -> Delta/1
  Subtract/1 -> Add/1
  Prsnt/1 -> Add/2

== system CM455A_Tauj0CfgAndUse/Tauj0CfgAndUse/Tauj0CfgAndUsePer1/Phase C Time Measurement/Delta >= 0 ==
  Prsnt : Inport
  Prev : Inport  Port=2
  Action Port : ActionPort  ActionType=then
  Subtract : Sum  Inputs=+-
  Delta : Outport
  wires:
  Subtract/1 -> Delta/1
  Prsnt/1 -> Subtract/1
  Prev/1 -> Subtract/2
